simulink model "Part1"  (R2020b)
settings: Solver=VariableStepAuto  StartTime=0.0  StopTime=80  RelTol=1e-3
settings Model: Creator=abdullah  LastModifiedBy=abdullah

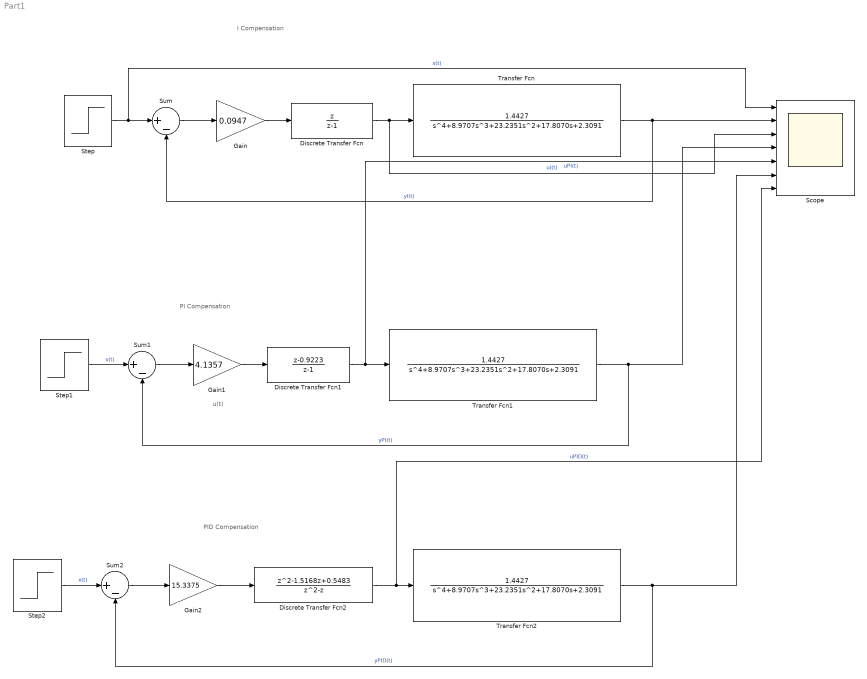
== system Part1 ==
  note: I Compensation
  note: PI Compensation
  note: u(t)
  note: PID Compensation
  Discrete Transfer Fcn : DiscreteTransferFcn  Numerator=[1 0]  Denominator=[1 -1]  SampleTime=0.5
  Discrete Transfer Fcn1 : DiscreteTransferFcn  Numerator=[1 -0.9223]  Denominator=[1 -1]  SampleTime=0.5
  Discrete Transfer Fcn2 : DiscreteTransferFcn  Numerator=[1 -1.5168 0.5483]  Denominator=[1 -1 0]  SampleTime=0.5
  Gain : Gain  Gain=0.0947
  Gain1 : Gain  Gain=4.1357
  Gain2 : Gain  Gain=15.3375
  Scope : Scope  NumInputPorts=7
  Step : Step  SampleTime=0
  Step1 : Step  SampleTime=0
  Step2 : Step  SampleTime=0
  Sum : Sum  Inputs=|+-
  Sum1 : Sum  Inputs=|+-
  Sum2 : Sum  Inputs=|+-
  Transfer Fcn : TransferFcn  Numerator=[1.4427]  Denominator=[1 8.9707 23.2351 17.8070 2.3091]
  Transfer Fcn1 : TransferFcn  Numerator=[1.4427]  Denominator=[1 8.9707 23.2351 17.8070 2.3091]
  Transfer Fcn2 : TransferFcn  Numerator=[1.4427]  Denominator=[1 8.9707 23.2351 17.8070 2.3091]
  wires:
  Gain/1 -> Discrete Transfer Fcn/1
  Discrete Transfer Fcn/1 -> Scope/3, Transfer Fcn/1  "uI(t)"
  Transfer Fcn/1 -> Sum/2, Scope/2  "yI(t)"
  Sum/1 -> Gain/1
  Step/1 -> Scope/1, Sum/1  "x(t)"
  Step1/1 -> Sum1/1  "x(t)"
  Discrete Transfer Fcn1/1 -> Scope/5, Transfer Fcn1/1  "uPI(t)"
  Transfer Fcn1/1 -> Scope/4, Sum1/2  "yPI(t)"
  Sum1/1 -> Gain1/1
  Gain1/1 -> Discrete Transfer Fcn1/1
  Step2/1 -> Sum2/1  "x(t)"
  Discrete Transfer Fcn2/1 -> Scope/7, Transfer Fcn2/1  "uPID(t)"
  Transfer Fcn2/1 -> Scope/6, Sum2/2  "yPID(t)"
  Sum2/1 -> Gain2/1
  Gain2/1 -> Discrete Transfer Fcn2/1
